simulink model "Nanogrid"  (R2026a)
settings: Solver=VariableStepAuto  StopTime=3
PreLoadFcn:
  | NanogridParam
undefined symbols (not defined in the file): baseLoad, bessSystem, bessVoltage, DiscIntNeverNeededParam, ee_sli_rtmsupport, gcbh, gflInverter, gfmInverter, nanoLoad, PV, PVInverter, ref, solar, solarInsolationChange, Ts
libraries: nesl_utility x51, eeGeneralControl x38, ee_lib x33, fl_lib x24, simulink x20, eeTransforms x13, slpidlib x8, nesl_utility_internal x4, sl_signal_attributes x4, sl_discontinuities x4, eeSinusoidalMeasurementV2 x3, batteryecm_lib x2
(part 4 of 6)

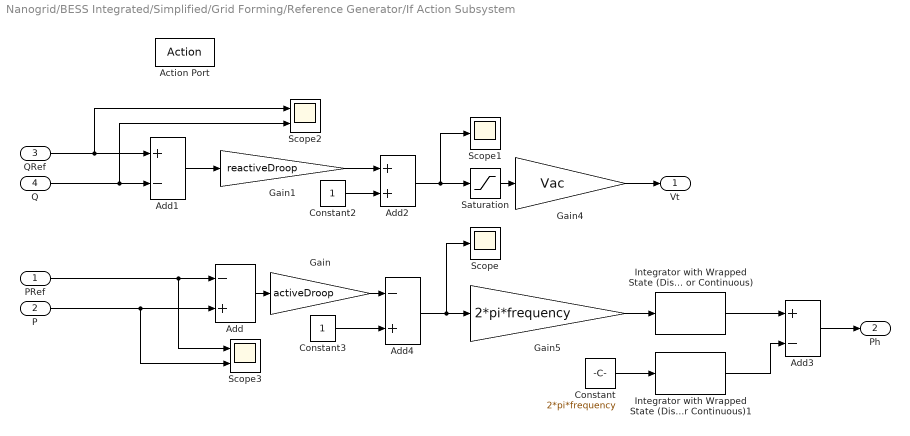
== system Nanogrid/BESS Integrated/Simplified/Grid Forming/Reference Generator/If Action Subsystem ==
  PRef : Inport
  P : Inport  Port=2
  QRef : Inport  Port=3
  Q : Inport  Port=4
  Action Port : ActionPort
  Add : Sum  Inputs=-+
  Add1 : Sum  Inputs=+-
  Add2 : Sum
  Add3 : Sum  Inputs=+-
  Add4 : Sum  Inputs=-+
  Constant : Constant  Value=2*pi*frequency  SampleTime=-1
  Constant2 : Constant
  Constant3 : Constant
  Gain : Gain  Gain=activeDroop
  Gain1 : Gain  Gain=reactiveDroop
  Gain4 : Gain  Gain=Vac
  Gain5 : Gain  Gain=2*pi*frequency
  Integrator with Wrapped State (Discrete or Continuous) : eeGeneralControl/Integrator with Wrapped State (Discrete or Continuous)  LabelModeActiveChoice=Discrete  WrappedStateUpperValue=2*pi  WrappedStateLowerValue=0  x0=0  Ts=-1
  Integrator with Wrapped State (Discrete or Continuous)1 : eeGeneralControl/Integrator with Wrapped State (Discrete or Continuous)  LabelModeActiveChoice=Discrete  WrappedStateUpperValue=2*pi  WrappedStateLowerValue=0  x0=0  Ts=-1
  Saturation : Saturate  UpperLimit=1.1  LowerLimit=0.9
  Scope : Scope
      settings: ActiveDisplayYMinimum=-1  ActiveDisplayYMaximum=1  DataLoggingVariableName=ScopeData2
  Scope1 : Scope
      settings: ActiveDisplayYMinimum=-1  ActiveDisplayYMaximum=1  DataLoggingVariableName=ScopeData3
  Scope2 : Scope  NumInputPorts=2
      settings: ActiveDisplayYMinimum=-1  ActiveDisplayYMaximum=1
  Scope3 : Scope  NumInputPorts=2
      settings: ActiveDisplayYMinimum=-1  ActiveDisplayYMaximum=1  DataLoggingVariableName=ScopeData2
  Vt : Outport
  Ph : Outport  Port=2
  wires:
  Add4/1 -> Scope/1, Gain5/1
  Gain/1 -> Add4/1
  Add1/1 -> Gain1/1
  Add2/1 -> Scope1/1, Saturation/1
  Gain5/1 -> Integrator with Wrapped State (Discrete or Continuous)/1
  Constant3/1 -> Add4/2
  Integrator with Wrapped State (Discrete or Continuous)/1 -> Add3/1
  Constant2/1 -> Add2/2
  Gain1/1 -> Add2/1
  Gain4/1 -> Vt/1
  QRef/1 -> Add1/1, Scope2/1
  Saturation/1 -> Gain4/1
  Add/1 -> Gain/1
  PRef/1 -> Add/1, Scope3/1
  Add3/1 -> Ph/1
  Constant/1 -> Integrator with Wrapped State (Discrete or Continuous)1/1
  Integrator with Wrapped State (Discrete or Continuous)1/1 -> Add3/2
  P/1 -> Add/2, Scope3/2
  Q/1 -> Add1/2, Scope2/2

== system Nanogrid/BESS Integrated/Simplified/Grid Forming/Reference Generator/If Action Subsystem1 ==
  PRef : Inport
  P : Inport  Port=2
  VRef : Inport  Port=3
  V : Inport  Port=4
  Action Port : ActionPort
  Add : Sum  Inputs=+-
  Add1 : Sum  Inputs=+-
  Add2 : Sum
  Add3 : Sum  Inputs=+-
  Add4 : Sum  Inputs=-+
  Constant2 : Constant
  Constant3 : Constant
  Constant4 : Constant  Value=0
  Gain : Gain  Gain=reactiveDroop
  Gain1 : Gain  Gain=activeDroop
  Gain4 : Gain  Gain=systemVoltage
  Gain5 : Gain  Gain=2*pi*systemFrequency
  Integrator with Wrapped State (Discrete or Continuous) : eeGeneralControl/Integrator with Wrapped State (Discrete or Continuous)  LabelModeActiveChoice=Discrete  WrappedStateUpperValue=2*pi  WrappedStateLowerValue=0  x0=0  Ts=-1
  Saturation : Saturate  UpperLimit=1.1  LowerLimit=0.9
  Vt : Outport
  Ph : Outport  Port=2
  wires:
  Add/1 -> Gain/1
  Constant4/1 -> Add3/2
  Add4/1 -> Gain5/1
  Gain/1 -> Add4/1
  Add1/1 -> Gain1/1
  Add2/1 -> Saturation/1
  Gain5/1 -> Integrator with Wrapped State (Discrete or Continuous)/1
  Constant3/1 -> Add4/2
  Integrator with Wrapped State (Discrete or Continuous)/1 -> Add3/1
  Constant2/1 -> Add2/2
  Gain1/1 -> Add2/1
  V/1 -> Add/2
  Gain4/1 -> Vt/1
  P/1 -> Add1/2
  VRef/1 -> Add/1
  PRef/1 -> Add1/1
  Add3/1 -> Ph/1
  Saturation/1 -> Gain4/1

== system Nanogrid/Solar Plant Integrated/Detailed/PV Plant & Controller/Controller/MPPT ==
  Qref : Inport
  ipv (A) : Inport  Port=2
  vdc (V) : Inport  Port=3
  Vabc : Inport  Port=4
  Iabc : Inport  Port=5
  Action Port : ActionPort  ActionPortLabel=if(u1 > 0)
  Solar PV Controller : Subsystem  LoadFcn=ee_sli_rtmsupport( 'loadfcn', gcbh );  mask(Solar PV Controller (Three-Phase)){L=filterInductance, frequency=frequency, iMax=iMaxPU, zBase=Vac^2/(plantRating*1000), mVAbase=plantRating*1000, VdcBase=baseVoltageDC, sampleTime=-1, Choice=Perturb and observe (P&O), Vdc=1100, delV=3, tSettling=1e-3, Kppll=100, Kipll=2000, initialPhase=0, Kpv=PV.controllerKpv, Kiv=PV.controllerKiv, Kdv=0, Kpicd=PV.controllerKpIc, Kiicd=PV.controllerKiIc, Kdicd=0, Kpicq=PV.controllerKpIc, Kiicq=PV.controllerKiIc, Kdicq=0}
      mask prompts: L "physmod:ee:library:comments:control:eeRenewablesControl:ACFilterInductanceH_MP"; frequency "physmod:ee:library:comments:control:eeRenewablesControl:SystemFrequencyHz_MP"; iMax "physmod:ee:library:comments:control:eeRenewablesControl:InverterCurrentLimitpu_MP"; zBase "physmod:ee:library:comments:control:eeRenewablesControl:BaseImpedanceACSideOhm_MP"; mVAbase "physmod:ee:library:comments:control:eeRenewablesControl:BaseMVA_MP"; VdcBase "physmod:ee:library:comments:control:eeRenewablesControl:DCBusBaseVoltageV_MP"; sampleTime "physmod:ee:library:comments:control:eeRenewablesControl:SampleTime1ForInherited_MP"; Choice "physmod:ee:library:comments:control:eeRenewablesControl:Algorithm_MP"; Vdc "physmod:ee:library:comments:control:eeRenewablesControl:InitialVoltageForMPPTV_MP"; delV "physmod:ee:library:comments:control:eeRenewablesControl:VoltageStepOfMPPTV_MP"; tSettling "physmod:ee:library:comments:control:eeRenewablesControl:SettlingTimeOfMPPTs_MP"; Kppll "physmod:ee:library:comments:control:eeRenewablesControl:ProportionalGain_MP"; Kipll "physmod:ee:library:comments:control:eeRenewablesControl:IntegralGain_MP"; initialPhase "physmod:ee:library:comments:control:eeRenewablesControl:InitialPhaseAngle_MP"; Kpv "physmod:ee:library:comments:control:eeRenewablesControl:ProportionalGain_MP"; Kiv "physmod:ee:library:comments:control:eeRenewablesControl:IntegralGain_MP"; Kdv "physmod:ee:library:comments:control:eeRenewablesControl:DerivativeGain_MP"; Kpicd "physmod:ee:library:comments:control:eeRenewablesControl:DaxisProportionalGain_MP"; Kiicd "physmod:ee:library:comments:control:eeRenewablesControl:DaxisIntegralGain_MP"; Kdicd "physmod:ee:library:comments:control:eeRenewablesControl:DaxisDerivativeGain_MP"; Kpicq "physmod:ee:library:comments:control:eeRenewablesControl:QaxisProportionalGain_MP"; Kiicq "physmod:ee:library:comments:control:eeRenewablesControl:QaxisIntegralGain_MP"; Kdicq "physmod:ee:library:comments:control:eeRenewablesControl:QaxisDerivativeGain_MP"
      mask help: physmod:ee:library:comments:control:eeRenewablesControl:PVGridFollowingController_MD
      mask init:
      | timeDomain = ee.mask.getSampleTimeDomain(sampleTime,gcb);
      | if sampleTime < 0 && sampleTime ~= -1            
      |     error(message('physmod:ee:library:MinusOneZeroOrPositive',getString(message('physmod:ee:library:comments:control:eeRenewablesControl:SampleTime1ForInherited_MP'))));            
      | end
      | if L <= 0            
      |     error(message('physmod:simscape:compiler:patterns:checks:GreaterThanZero',getString(message('physmod:ee:library:comments:control:eeRenewablesControl:ACFilterInductanceH_MP'))));            
      | end
      | if VdcBase <= 0            
      |     error(message('physmod:simscape:compiler:patterns:checks:GreaterThanZero',getString(message('physmod:ee:library:comments:control:eeRenewablesControl:DCBusBaseVoltageV_MP'))));            
      | end
      | if delV <= 0            
      |     error(message('physmod:simscape:compiler:patterns:checks:GreaterThanZero',getString(message('physmod:ee:library:comments:control:eeRenewablesControl:VoltageStepOfMPPTV_MP'))));            
      | end
      | if tSettling <= 0            
      |     error(message('physmod:simscape:compiler:patterns:checks:GreaterThanZero',getString(message('physmod:ee:library:comments:control:eeRenewablesControl:SettlingTimeOfMPPTs_MP'))));            
      | end
      | if zBase <= 0            
      |     error(message('physmod:simscape:compiler:patterns:checks:GreaterThanZero',getString(message('physmod:ee:library:comments:control:eeRenewablesControl:BaseImpedanceACSideOhm_MP'))));            
      | end
      | if iMax <= 0            
      |     error(message('physmod:simscape:compiler:patterns:checks:GreaterThanZero',getString(message('physmod:ee:library:comments:control:eeRenewablesControl:InverterCurrentLimitpu_MP'))));            
      | end
      | if frequency <= 0            
      |     error(message('physmod:simscape:compiler:patterns:checks:GreaterThanZero',getString(message('physmod:ee:library:comments:control:eeRenewablesControl:SystemFrequencyHz_MP'))));            
      | end
      settings: CopyFcn=ee_sli_rtmsupport( 'copyfcn', gcbh );  DeleteFcn=ee_sli_rtmsupport( 'deletefcn', gcbh );  ModelCloseFcn=ee_sli_rtmsupport( 'modelclosefcn', gcbh );  PostSaveFcn=ee_sli_rtmsupport( 'postsavefcn', gcbh );  PreCopyFcn=ee_sli_rtmsupport( 'precopyfcn', gcbh );  OpenFcn=ee_sli_rtmsupport( 'openfcn', gcbh );  CloseFcn=ee_sli_rtmsupport( 'closefcn', gcbh );  PreDeleteFcn=ee_sli_rtmsupport( 'predeletefcn', gcbh );
      mask Help: web(nesl_help(gcbh))
      mask TypeOptions sampleTime: Current_controller/SystemSampleTime | DC voltage controller & current reference/SystemSampleTime
      mask TypeOptions Choice: Variant Subsystem/LabelModeActiveChoice
      mask DialogControl Container4 Prompt: physmod:ee:library:comments:control:eeRenewablesControl:General_Tab
      mask DialogControl L Prompt: AC filter inductance (H)
      mask DialogControl frequency Prompt: System frequency (Hz)
      mask DialogControl iMax Prompt: Inverter current limit (pu)
      mask DialogControl zBase Prompt: Base impedance on AC side (Ohm)
      mask DialogControl mVAbase Prompt: Base power on AC side (V*A)
      mask DialogControl VdcBase Prompt: DC bus base voltage (V)
      mask DialogControl sampleTime Prompt: Sample time (-1 for inherited)
      mask DialogControl Container5 Prompt: physmod:ee:library:comments:control:eeRenewablesControl:MPPT_Tab
      mask DialogControl Choice Prompt: Algorithm
      mask DialogControl Vdc Prompt: Initial voltage for MPPT (V)
      mask DialogControl delV Prompt: Voltage step of MPPT (V)
      mask DialogControl tSettling Prompt: Settling time of MPPT (s)
      mask DialogControl Container6 Prompt: physmod:ee:library:comments:control:eeRenewablesControl:PLL_Tab
      mask DialogControl Kppll Prompt: Proportional gain
      mask DialogControl Kipll Prompt: Integral gain
      mask DialogControl initialPhase Prompt: Initial phase angle (deg)
      mask DialogControl Container7 Prompt: physmod:ee:library:comments:control:eeRenewablesControl:VoltageController_Tab
      mask DialogControl Kpv Prompt: Proportional gain
      mask DialogControl Kiv Prompt: Integral gain
      mask DialogControl Kdv Prompt: Derivative gain
      mask DialogControl Container8 Prompt: physmod:ee:library:comments:control:eeRenewablesControl:CurrentController_Tab
      mask DialogControl Kpicd Prompt: D-axis proportional gain
      mask DialogControl Kiicd Prompt: D-axis integral gain
      mask DialogControl Kdicd Prompt: D-axis derivative gain
      mask DialogControl Kpicq Prompt: Q-axis proportional gain
      mask DialogControl Kiicq Prompt: Q-axis integral gain
      mask DialogControl Kdicq Prompt: Q-axis derivative gain
      mask Display: ee.mask.drawPVcontroller;
  mabc : Outport
  wires:
  ipv (A)/1 -> Solar PV Controller/2(ipv (A))
  Iabc/1 -> Solar PV Controller/5(iabc (pu))
  Vabc/1 -> Solar PV Controller/4(vabc (pu))
  vdc (V)/1 -> Solar PV Controller/3(vdc (V))
  Qref/1 -> Solar PV Controller/1(Qref (pu))
  Solar PV Controller/1(vabcRef (pu)) -> mabc/1

== system Nanogrid/Solar Plant Integrated/Detailed/PV Plant & Controller/Controller/Power Reference ==
  Iabc : Inport
  Vabc : Inport  Port=2
  PRef : Inport  Port=3
  QRef : Inport  Port=4
  Action Port : ActionPort  ActionPortLabel=else
  Power Reference Controller : Subsystem  mask(Power Reference Controller){frequency=frequency, P=Real power, MVA=plantRating*1000, zbase=Vac^2/plantRating, L=filterInductance, Imax=iMaxPU, Td=1e-3, Kpic=1.5, Kiic=10, Kd=0, kpPLL=40, kiPLL=1000, kdPLL=0}
      mask prompts: frequency "Frequency (Hz)"; P "Priority mode"; MVA "Base Power (V*A)"; zbase "Base Impedance (Ohm)"; L "Filter Inductance (H)"; Imax "Inverter current limit (pu)"; Td "Sensor time delay (s)"; Kpic "Proportional gain"; Kiic "Integral gain"; Kd "Derevative gain"; kpPLL "Proportional gain"; kiPLL "Integral gain"; kdPLL "Derevative gain"
      mask help: This block receives active and reactive power references for the converter based on system requirements or higher-level control commands. It ensures that the converter operates according to desired power setpoints, supporting grid services such as frequency regulation, voltage support, and power dispatch
      settings: CopyFcn=set_param(gcbh,'LinkStatus','none');
      mask TypeOptions P: Real power  | Reactive power
      mask DialogControl Container4 Prompt: General
      mask DialogControl Container5 Prompt: Current Controller
      mask DialogControl Container5_copy Prompt: PLL
  mabc : Outport
  wires:
  QRef/1 -> Power Reference Controller/4(Qref)
  PRef/1 -> Power Reference Controller/3(Pref)
  Power Reference Controller/1(mabc) -> mabc/1
  Vabc/1 -> Power Reference Controller/2(Vabc)
  Iabc/1 -> Power Reference Controller/1(Iabc)

== system Nanogrid/Solar Plant Integrated/Detailed/PV Plant & Controller/PV Plant/Converter ==
  mabc : Inport
  Average : Subsystem  VariantControl=Average
  Switching : Subsystem  VariantControl=Switching
  + : PMIOPort  Side=Left
  - : PMIOPort  Port=2  Side=Left
  ~ : PMIOPort  Port=3  Side=Right

== system Nanogrid/Solar Plant Integrated/Detailed/PV Plant & Controller/Sensor Dynamics/Current Measurement ==
  u : Inport
  Lead-Lag (Discrete or Continuous) : eeGeneralControl/Lead-Lag (Discrete or Continuous)  T1=0  T2=PV.controllerTSensor  B=inf  A=-inf  init_option=Inherited from block input  x0=0  Ts=Ts
  V : Outport
  wires:
  u/1 -> Lead-Lag (Discrete or Continuous)/1
  Lead-Lag (Discrete or Continuous)/1 -> V/1

== system Nanogrid/Solar Plant Integrated/Detailed/PV Plant & Controller/Sensor Dynamics/Voltage Measurement ==
  u : Inport
  Lead-Lag (Discrete or Continuous) : eeGeneralControl/Lead-Lag (Discrete or Continuous)  T1=0  T2=PV.controllerTSensor  B=inf  A=-inf  init_option=Inherited from block input  x0=0  Ts=Ts
  I : Outport
  wires:
  u/1 -> Lead-Lag (Discrete or Continuous)/1
  Lead-Lag (Discrete or Continuous)/1 -> I/1

== system Nanogrid/BESS Integrated/Detailed/BESS Controller/Grid Following/Reference Current/Current limits ==
  Imax : Inport
  iqref : Inport  Port=2
  idref : Inport  Port=3
  Constant8 : Constant  Value=0
  Constant9 : Constant  Value=0
  Scope : Scope
      settings: ActiveDisplayYMinimum=-0.14399  ActiveDisplayYMaximum=1.29587  DataLoggingVariableName=ScopeData3
  Scope1 : Scope
      settings: ActiveDisplayYMinimum=-0.13655  ActiveDisplayYMaximum=1.22893  DataLoggingVariableName=ScopeData4
  Sqrt : Sqrt
  Sqrt1 : Sqrt
  Square{1..4} (4 alike) : Math  Operator=square
  Step2 : Step  Time=0.01  SampleTime=Ts
  Step3 : Step  Time=0.01  SampleTime=Ts
  Sum6 : Sum  Inputs=|+-
  Sum9 : Sum  Inputs=|+-
  Switch1 : Switch  Threshold=.01  SaturateOnIntegerOverflow=off  InputSameDT=off
  Switch2 : Switch  Threshold=.01  SaturateOnIntegerOverflow=off  InputSameDT=off
  iubq : Outport
  iubd : Outport  Port=2
  wires:
  idref/1 -> Square4/1
  Sqrt1/1 -> iubq/1, Scope1/1
  Imax/1 -> Square1/1, Square3/1
  Sqrt/1 -> iubd/1, Scope/1
  Constant9/1 -> Switch2/3
  Square4/1 -> Sum9/2
  Constant8/1 -> Switch1/3
  Square2/1 -> Sum6/2
  Sum6/1 -> Switch1/1
  Square3/1 -> Sum9/1
  iqref/1 -> Square2/1
  Switch1/1 -> Sqrt/1
  Square1/1 -> Sum6/1
  Switch2/1 -> Sqrt1/1
  Step2/1 -> Switch1/2
  Step3/1 -> Switch2/2
  Sum9/1 -> Switch2/1

== system Nanogrid/BESS Integrated/Detailed/BESS Controller/Grid Following/Reference Current/Refernce id generation ==
  V_mag : Inport
  del f : Inport  Port=2
  ubid : Inport  Port=3
  PRef : Inport  Port=4
  Divide : Product  Inputs=/*
  Gain6 : Gain  Gain=-1
  P/Q Priority : Switch  Criteria=u2 ~= 0  SaturateOnIntegerOverflow=off  InputSameDT=off
  Priority Mode : Constant  Value=P-2
  Saturation Dynamic2 : simulink/Discontinuities/Saturation Dynamic  OutMin=[]  OutMax=[]  OutDataTypeStr=Inherit: Same as second input  OutDataType=fixdt(1, 16)  OutScaling=2^-10  DoSatur=off
  Saturation1 : Saturate  UpperLimit=Imax  LowerLimit=-Imax
  Scope : Scope
      settings: ActiveDisplayYMinimum=-1  ActiveDisplayYMaximum=1
  Scope1 : Scope
      settings: ActiveDisplayYMinimum=-0.68622  ActiveDisplayYMaximum=0.07625  DataLoggingVariableName=ScopeData2
  Sum : Sum  Inputs=|++
  droop m_p : Gain  Gain=mp/MVA
  ubid1 : InportShadow  Port=3
  id_ref : Outport
  wires:
  del f/1 -> droop m_p/1
  Divide/1 -> Saturation Dynamic2/2, Saturation1/1
  V_mag/1 -> Divide/1
  P/Q Priority/1 -> id_ref/1, Scope/1
  ubid1/1 -> Gain6/1
  Saturation1/1 -> P/Q Priority/1
  Priority Mode/1 -> P/Q Priority/2
  PRef/1 -> Sum/2
  Saturation Dynamic2/1 -> P/Q Priority/3, Scope1/1
  Gain6/1 -> Saturation Dynamic2/3
  ubid/1 -> Saturation Dynamic2/1
  Sum/1 -> Divide/2
  droop m_p/1 -> Sum/1

== system Nanogrid/BESS Integrated/Detailed/BESS Controller/Grid Following/Reference Current/Refernce iq generation ==
  ubiq : Inport
  V_ref : Inport  Port=2
  V_mag : Inport  Port=3
  LVRT_iq : Inport  Port=4
  Q_ref : Inport  Port=5
  Divide1 : Product  Inputs=*/
  Gain : Gain  Gain=-1
  Gain1 : Gain  Gain=-1
  Gain7 : Gain  Gain=-1
  LVRT Priority : Switch  Threshold=.9  SaturateOnIntegerOverflow=off  InputSameDT=off
  P/Q Priority : Switch  Criteria=u2 ~= 0  SaturateOnIntegerOverflow=off  InputSameDT=off
  Priority Mode : Constant  Value=P-2
  Saturation Dynamic : simulink/Discontinuities/Saturation Dynamic  OutMin=[]  OutMax=[]  OutDataTypeStr=Inherit: Same as second input  OutDataType=fixdt(1, 16)  OutScaling=2^-10  DoSatur=off
  Saturation2 : Saturate  UpperLimit=1  LowerLimit=-1
  Saturation3 : Saturate  UpperLimit=Imax  LowerLimit=-Imax
  Sum : Sum  Inputs=|++
  Sum1 : Sum  Inputs=|-+
  droop m_v : Gain  Gain=mv
  ubiq1 : InportShadow
  iq_ref : Outport
  wires:
  Gain/1 -> iq_ref/1
  V_mag/1 -> Sum1/2, Divide1/2, LVRT Priority/2
  Q_ref/1 -> Sum/1
  Sum/1 -> Divide1/1
  droop m_v/1 -> Sum/2
  ubiq1/1 -> Gain7/1
  LVRT_iq/1 -> Saturation2/1
  V_ref/1 -> Sum1/1
  Gain7/1 -> Saturation Dynamic/3
  Saturation Dynamic/1 -> P/Q Priority/1
  Divide1/1 -> Saturation3/1, Saturation Dynamic/2
  Priority Mode/1 -> P/Q Priority/2
  Saturation3/1 -> P/Q Priority/3
  Saturation2/1 -> Gain1/1
  ubiq/1 -> Saturation Dynamic/1
  Gain1/1 -> LVRT Priority/3
  P/Q Priority/1 -> LVRT Priority/1
  Sum1/1 -> droop m_v/1
  LVRT Priority/1 -> Gain/1

== system Nanogrid/BESS Integrated/Detailed/BESS Controller/Grid Forming/Current Limiting/CurrentLimitingMethod ==
  Igd : Inport
  Igq : Inport  Port=2
  currentLimitAndVirtual : Subsystem  VariantControl=both
  currentSaturation : Subsystem  VariantControl=ctSat
  virtualImpedance : Subsystem  VariantControl=virimp
  delVd : Outport
  delVq : Outport  Port=2
  Idmax : Outport  Port=3
  Iqmax : Outport  Port=4

== system Nanogrid/BESS Integrated/Detailed/BESS Controller/Grid Forming/Grid Voltage Reactive Power Support/Modifying Active Power Reference ==
  PrefInput : Inport
  Vd : Inport  Port=2
  Igd : Inport  Port=3
  Igq : Inport  Port=4
  AND : Logic  IconShape=distinctive  AllPortsSameDT=off  OutDataTypeStr=boolean
  Abs : Abs  SaturateOnIntegerOverflow=off
  Compare To Constant : simulink/Logic and Bit Operations/Compare To Constant  relop=>=  const=0.95  OutDataTypeStr=boolean
  Computing New Active Power Ref : Subsystem
  Math Function1 : Math  Operator=hypot
  Power Sign : Signum
  Product : Product
  Relay : Relay  OnSwitchValue=40%maxVICurrentLimit*0.96  OffSwitchValue=1
  Scope : Scope
  Scope1 : Scope
  Scope2 : Scope
  Switch : Switch  Criteria=u2 > Threshold  SaturateOnIntegerOverflow=off  InputSameDT=off
  Pref : Outport
  wires:
  Compare To Constant/1 -> AND/1
  AND/1 -> Switch/2
  Relay/1 -> AND/2, Scope1/1
  Product/1 -> Pref/1
  Power Sign/1 -> Product/2
  Abs/1 -> Product/1
  Switch/1 -> Abs/1
  Igq/1 -> Math Function1/1, Computing New Active Power Ref/1(Iq)
  Igd/1 -> Math Function1/2
  PrefInput/1 -> Switch/3, Power Sign/1
  Vd/1 -> Compare To Constant/1, Computing New Active Power Ref/2(Vd)
  Math Function1/1 -> Relay/1, Scope2/1  "Is"
  Computing New Active Power Ref/1(Pref) -> Scope/1, Switch/1

== system Nanogrid/BESS Integrated/Detailed/BESS Controller/Grid Forming/Grid Voltage Reactive Power Support/Modifying Reactive Power Reference ==
  Vgd : Inport
  Vgq : Inport  Port=2
  Qref : Inport  Port=3
  Pref : Inport  Port=4
  Changing the Power Reference : Subsystem
  Hysteresis : Subsystem
  Math Function : Math  Operator=hypot
  Merge : Merge
  Merge1 : Merge
  NOT : Logic  Operator=NOT  IconShape=distinctive  AllPortsSameDT=off  OutDataTypeStr=boolean
  Not Altering the Power Reference : Subsystem
  Scope : Scope
  PrefNew : Outport
  QrefNew : Outport  Port=2
  wires:
  [Qref] -> Changing the Power Reference/4(Qref)
  [Pref] -> Changing the Power Reference/3(Pref)
  Merge/1 -> PrefNew/1
  Merge1/1 -> QrefNew/1
  Pref/1 -> [Pref], Not Altering the Power Reference/1(Pref)
  Vgq/1 -> Math Function/2
  Changing the Power Reference/2(Qrefv) -> Merge1/1
  [Vd] -> Changing the Power Reference/2(Vd)
  Hysteresis/1(LVFlag) -> NOT/1, Changing the Power Reference/Enable, Scope/1
  Qref/1 -> [Qref], Not Altering the Power Reference/2(Qref)
  NOT/1 -> Not Altering the Power Reference/Enable
  Changing the Power Reference/1(Prefv) -> Merge/1
  Not Altering the Power Reference/1(Prefv) -> Merge/2
  [Vs] -> Changing the Power Reference/1(Vs)
  Math Function/1 -> [Vs], Hysteresis/1(Vs)
  Not Altering the Power Reference/2(Qrefv) -> Merge1/2
  Vgd/1 -> Math Function/1, [Vd]

== system Nanogrid/BESS Integrated/Detailed/BESS Controller/Grid Forming/Measurement/Frequency Measurement ==
  Vabc : Inport
  Convert To PU : Gain  Gain=1/powerFreq
  Frequency Measurement : Subsystem  TreatAsAtomicUnit=on  SystemSampleTime=sampleTime  mask{initialFrequency=powerFreq, sampleTime=activePowerSampleTime}
      mask prompts: initialFrequency "Initial frequency in Hz"; sampleTime "Sample time in sec"
      mask DialogControl Container7 Prompt: General
  Low-Pass Filter : eeGeneralControl/Low-Pass Filter (Discrete or Continuous)  K=1  T=freqMeasTimeConst  B=inf  A=-inf  init_option=Inherited from block input  x0=0  Ts=-1
  freq : Outport
  wires:
  Vabc/1 -> Frequency Measurement/1(abc)
  Convert To PU/1 -> freq/1
  Frequency Measurement/1(Freq) -> Low-Pass Filter/1
  Low-Pass Filter/1 -> Convert To PU/1  "Freq"

== system Nanogrid/BESS Integrated/Detailed/BESS Controller/Grid Forming/Measurement/abc2dq ==
  Igabc : Inport
  Angle : Inport  Port=2
  Vgabc : Inport  Port=3
  Supply Current to dq : Subsystem
  Supply Voltage  to dq1 : Subsystem
  Vgd : Outport
  Vgq : Outport  Port=2
  Igd : Outport  Port=3
  Igq : Outport  Port=4
  wires:
  Supply Voltage  to dq1/2(Vgq) -> Vgq/1  "Vgq"
  Supply Voltage  to dq1/1(Vgd) -> Vgd/1  "Vgd"
  Supply Current to dq/2(Igq) -> Igq/1  "Iq"
  Supply Current to dq/1(Igd) -> Igd/1  "Id"
  Igabc/1 -> Supply Current to dq/1(abc)
  Vgabc/1 -> Supply Voltage  to dq1/2(abc)
  Angle/1 -> Supply Current to dq/2(Angle), Supply Voltage  to dq1/1(Angle)

== system Nanogrid/BESS Integrated/Detailed/BESS Controller/Grid Forming/Power Control/ActivePowerControl ==
  Pref : Inport
  Pmeas : Inport  Port=2
  fref : Inport  Port=3
  cntrlflag : Inport  Port=4
  fgrid : Inport  Port=5
  droopControl : Subsystem  VariantControl=droop
  vsmControl : Subsystem  VariantControl=vsm
  Theta : Outport
  w : Outport  Port=2

== system Nanogrid/BESS Integrated/Detailed/BESS Controller/Grid Forming/Power Control/ReactiveControl ==
  note: Vs-delV
  CntrlFlag : Inport
  Qref : Inport  Port=2
  Qmeas : Inport  Port=3
  Vgdmeas : Inport  Port=4
  Vref : Inport  Port=5
  Constant2 : Constant  Value=0
  Saturation1 : Saturate  UpperLimit=(dcBusVoltage/2)/(sqrt(2/3)*girdLineVoltage)  LowerLimit=-(dcBusVoltage/2)/(sqrt(2/3)*girdLineVoltage)
  Scope : Scope
      settings: ActiveDisplayYMinimum=-1  ActiveDisplayYMaximum=1  DataLoggingVariableName=ScopeData20
  Voltage  Reference Selection : Subsystem
  Vmd : Outport
  Vmq : Outport  Port=2
  wires:
  Vgdmeas/1 -> Voltage  Reference Selection/5(Vgdmeas)
  Vref/1 -> Voltage  Reference Selection/4(Vref)
  Qmeas/1 -> Voltage  Reference Selection/3(Qmeas)
  Qref/1 -> Voltage  Reference Selection/2(Qref)
  CntrlFlag/1 -> Voltage  Reference Selection/1(cntrlflag)
  Saturation1/1 -> Vmd/1, Scope/1
  Constant2/1 -> Vmq/1
  Voltage  Reference Selection/1(Vd) -> Saturation1/1  "Q"

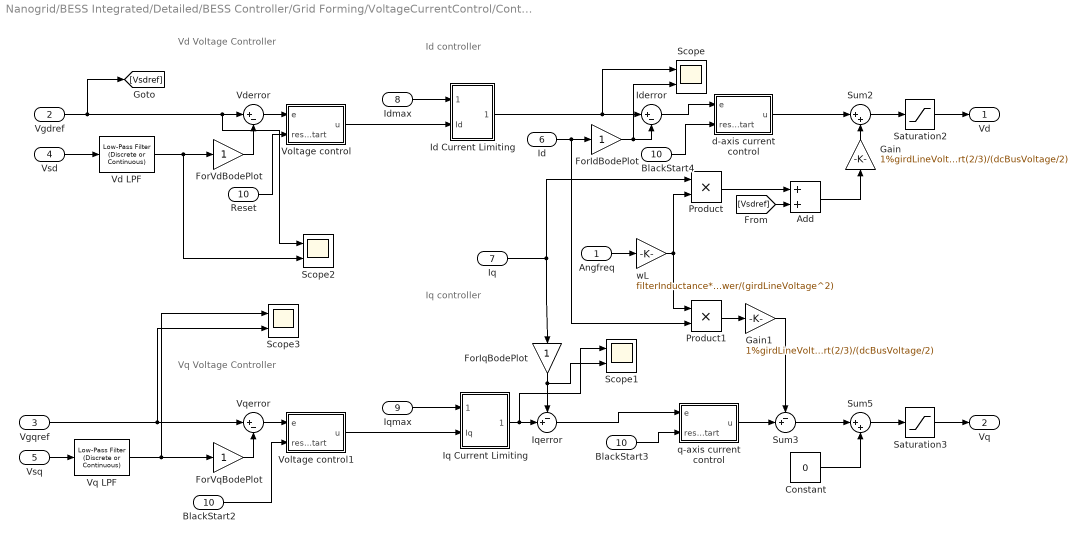
== system Nanogrid/BESS Integrated/Detailed/BESS Controller/Grid Forming/VoltageCurrentControl/Controller ==
  note: Vq Voltage Controller
  note: Iq controller
  note: Vd Voltage Controller
  note: Id controller
  Angfreq : Inport
  Vgdref : Inport  Port=2
  Vgqref : Inport  Port=3
  Vsd : Inport  Port=4
  Vsq : Inport  Port=5
  Id : Inport  Port=6
  Iq : Inport  Port=7
  Idmax : Inport  Port=8
  Iqmax : Inport  Port=9
  Reset : Inport  Port=10
  Add : Sum
  BlackStart2 : InportShadow  Port=10
  BlackStart3 : InportShadow  Port=10
  BlackStart4 : InportShadow  Port=10
  Constant : Constant  Value=0  SampleTime=currentControlTs
  ForIdBodePlot : Gain
  ForIqBodePlot : Gain
  ForVdBodePlot : Gain
  ForVqBodePlot : Gain
  Gain : Gain  Gain=1%girdLineVoltage*sqrt(2/3)/(dcBusVoltage/2)
  Gain1 : Gain  Gain=1%girdLineVoltage*sqrt(2/3)/(dcBusVoltage/2)
  Id Current Limiting : Subsystem
  Iderror : Sum  Inputs=|+-
  Iq Current Limiting : Subsystem
  Iqerror : Sum  Inputs=-+|
  Product : Product
  Product1 : Product
  Saturation2 : Saturate  UpperLimit=4  LowerLimit=-3
  Saturation3 : Saturate  UpperLimit=3  LowerLimit=-3
  Scope{,1..3} (4 alike) : Scope  NumInputPorts=2
      Scope settings: ActiveDisplayYMinimum=-0.33488  ActiveDisplayYMaximum=2.03721
      Scope2 settings: ActiveDisplayYMinimum=-0.14129  ActiveDisplayYMaximum=1.2716
  Sum2 : Sum  Inputs=|++
  Sum3 : Sum  Inputs=-+|
  Sum5 : Sum  Inputs=|++
  Vd LPF : eeGeneralControl/Low-Pass Filter (Discrete or Continuous)  K=1  T=vdvqLPFTimeConst  B=inf  A=-inf  init_option=Specify as parameter  x0=0  Ts=voltControlTs
  Vderror : Sum  Inputs=|+-
  Voltage control : Subsystem
  Voltage control1 : Subsystem
  Vq LPF : eeGeneralControl/Low-Pass Filter (Discrete or Continuous)  K=1  T=vdvqLPFTimeConst  B=inf  A=-inf  init_option=Inherited from block input  x0=0  Ts=voltControlTs
  Vqerror : Sum  Inputs=|+-
  d-axis current control : Subsystem
  q-axis current control : Subsystem
  wL : Gain  Gain=filterInductance*power/(girdLineVoltage^2)
  Vd : Outport  VectorParamsAs1DForOutWhenUnconnected=off
  Vq : Outport  Port=2  VectorParamsAs1DForOutWhenUnconnected=off
  wires:
  Vgdref/1 -> [Vsdref], Vderror/1, Scope2/1
  BlackStart4/1 -> d-axis current control/2(resetBlackStart)
  BlackStart3/1 -> q-axis current control/2(resetBlackStart)
  BlackStart2/1 -> Voltage control1/2(resetBlackStart)
  Reset/1 -> Voltage control/2(resetBlackStart)
  Vq LPF/1 -> ForVqBodePlot/1, Scope3/1
  Vd LPF/1 -> ForVdBodePlot/1, Scope2/2
  Id Current Limiting/1(Idref) -> Iderror/1, Scope/1
  ForIqBodePlot/1 -> Iqerror/1, Scope1/2
  ForIdBodePlot/1 -> Iderror/2, Scope/2
  ForVqBodePlot/1 -> Vqerror/2
  ForVdBodePlot/1 -> Vderror/2
  Vsd/1 -> Vd LPF/1
  Voltage control1/1(u) -> Iq Current Limiting/2(Iq)
  Iq Current Limiting/1(Iqref) -> Iqerror/2, Scope1/1
  Idmax/1 -> Id Current Limiting/1(Imax)
  Voltage control/1(u) -> Id Current Limiting/2(Id)
  Gain/1 -> Sum2/2
  Add/1 -> Gain/1
  [Vsdref] -> Add/2
  Gain1/1 -> Sum3/1
  Vqerror/1 -> Voltage control1/1(e)
  Vgqref/1 -> Vqerror/1, Scope3/2
  Iqmax/1 -> Iq Current Limiting/1(Imax)
  Vderror/1 -> Voltage control/1(e)
  Id/1 -> ForIdBodePlot/1, Product1/2
  Vsq/1 -> Vq LPF/1
  Sum5/1 -> Saturation3/1
  Sum3/1 -> Sum5/1
  q-axis current control/1(u) -> Sum3/2
  Sum2/1 -> Saturation2/1
  d-axis current control/1(u) -> Sum2/1
  Product/1 -> Add/1
  Product1/1 -> Gain1/1
  Saturation2/1 -> Vd/1
  Saturation3/1 -> Vq/1
  Iderror/1 -> d-axis current control/1(e)
  Constant/1 -> Sum5/2
  Angfreq/1 -> wL/1
  Iq/1 -> Product/1, ForIqBodePlot/1
  wL/1 -> Product/2, Product1/1
  Iqerror/1 -> q-axis current control/1(e)

== system Nanogrid/BESS Integrated/Detailed/BESS Controller/Grid Forming/VoltageCurrentControl/Modulation Signal ==
  Vd : Inport
  Vq : Inport  Port=2
  Angle : Inport  Port=3
  Constant : Constant  Value=0
  Inverse Park Transform : eeTransforms/Inverse Park Transform  AxisAlignment=D-axis  PowerInvariant=off
  Mux1 : Mux  Inputs=3
  Saturation2 : Saturate  UpperLimit=1  LowerLimit=-1
  Scope : Scope  NumInputPorts=2
      settings: DataLoggingVariableName=ScopeData9
  Scope1 : Scope
  mabc : Outport  VectorParamsAs1DForOutWhenUnconnected=off
  wires:
  Vq/1 -> Mux1/2, Scope/2
  Vd/1 -> Mux1/1, Scope/1
  Constant/1 -> Mux1/3
  Saturation2/1 -> mabc/1
  Angle/1 -> Inverse Park Transform/2, Scope1/1
  Mux1/1 -> Inverse Park Transform/1
  Inverse Park Transform/1 -> Saturation2/1

== system Nanogrid/BESS Integrated/Detailed/BESS Plant/Converter/Switching/Pulse Generation ==
  G : Inport
  Constant : Constant  Value=5
  Subtract : Sum  Inputs=-+
  G1 : Outport  VectorParamsAs1DForOutWhenUnconnected=off
  G2 : Outport  Port=2  VectorParamsAs1DForOutWhenUnconnected=off
  wires:
  G/1 -> Subtract/1, G1/1
  Constant/1 -> Subtract/2
  Subtract/1 -> G2/1

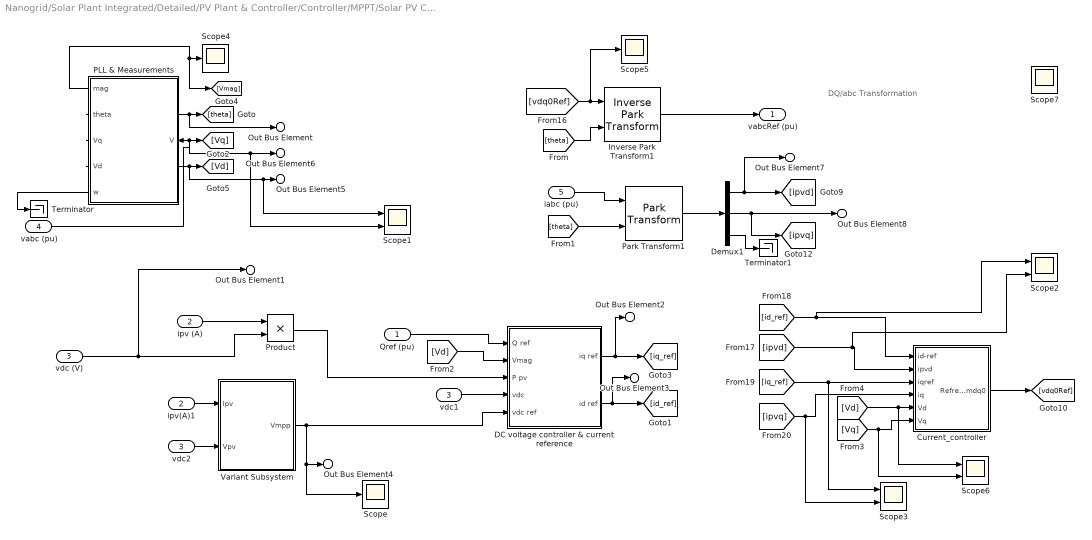
== system Nanogrid/Solar Plant Integrated/Detailed/PV Plant & Controller/Controller/MPPT/Solar PV Controller ==
  note: DQ/abc Transformation
  Qref (pu) : Inport
  ipv (A) : Inport  Port=2
  vdc (V) : Inport  Port=3
  vabc (pu) : Inport  Port=4
  iabc (pu) : Inport  Port=5
  Current_controller : Subsystem  SystemSampleTime=sampleTime
  DC voltage controller & current reference : Subsystem  SystemSampleTime=sampleTime
  Demux1 : Demux  Outputs=3
  Inverse Park Transform1 : eeTransforms/Inverse Park Transform  AxisAlignment=Q-axis  PowerInvariant=off
  PLL & Measurements : Subsystem
  Park Transform1 : eeTransforms/Park Transform  AxisAlignment=Q-axis  PowerInvariant=off
  Product : Product
  Scope{,4..5,7} (4 alike) : Scope
      Scope settings: ActiveDisplayYMinimum=719.47133  ActiveDisplayYMaximum=1441.72759  DataLoggingVariableName=ScopeData5
      Scope4 settings: ActiveDisplayYMinimum=-1  ActiveDisplayYMaximum=1
      Scope5 settings: ActiveDisplayYMinimum=-1  ActiveDisplayYMaximum=1
      Scope7 settings: DataLoggingVariableName=ScopeData43
  Scope{1..3,6} (4 alike) : Scope  NumInputPorts=2
      Scope1 settings: ActiveDisplayYMinimum=-0.005645300550064819  ActiveDisplayYMaximum=1.3041540601269743  DataLoggingVariableName=ScopeData6
      Scope2 settings: ActiveDisplayYMinimum=-0.14999999999999997  ActiveDisplayYMaximum=1.3499999999999999
      Scope3 settings: ActiveDisplayYMinimum=-0.016333965026179058  ActiveDisplayYMaximum=0.0079163760872077091
      Scope6 settings: ActiveDisplayYMinimum=-1  ActiveDisplayYMaximum=1  DataLoggingVariableName=ScopeData6
  Terminator : Terminator
  Terminator1 : Terminator
  Variant Subsystem : Subsystem  Variant=on  VariantControlMode=label  LabelModeActiveChoice=Perturb and observe (P&O)
  ipv(A)1 : InportShadow  Port=2
  vdc1 : InportShadow  Port=3
  vdc2 : InportShadow  Port=3
  vabcRef (pu) : Outport
  Out Bus Element : Outport  Port=2  PortName=visualization  Element=theta [rad]
  Out Bus Element1 : Outport  Port=2  PortName=visualization  Element=vdc [Volts]
  Out Bus Element2 : Outport  Port=2  PortName=visualization  Element=iq ref [pu]
  Out Bus Element3 : Outport  Port=2  PortName=visualization  Element=id ref [pu]
  Out Bus Element4 : Outport  Port=2  PortName=visualization  Element=vdc ref [Volts]
  Out Bus Element5 : Outport  Port=2  PortName=visualization  Element=Vd [pu]
  Out Bus Element6 : Outport  Port=2  PortName=visualization  Element=Vq [pu]
  Out Bus Element7 : Outport  Port=2  PortName=visualization  Element=id [pu]
  Out Bus Element8 : Outport  Port=2  PortName=visualization  Element=iq [pu]
  wires:
  PLL & Measurements/2(theta) -> [theta], Out Bus Element/1
  ipv(A)1/1 -> Variant Subsystem/1(Ipv)
  vdc2/1 -> Variant Subsystem/2(Vpv)
  ipv (A)/1 -> Product/1
  PLL & Measurements/5(w) -> Terminator/1
  Variant Subsystem/1(Vmpp) -> DC voltage controller & current reference/5(vdc ref), Scope/1, Out Bus Element4/1
  vdc1/1 -> DC voltage controller & current reference/4(vdc)
  vabc (pu)/1 -> PLL & Measurements/1(V)
  PLL & Measurements/4(Vd) -> [Vd], Scope1/1, Out Bus Element5/1
  PLL & Measurements/1(mag) -> Scope4/1, [Vmag]
  PLL & Measurements/3(Vq) -> [Vq], Scope1/2, Out Bus Element6/1
  Product/1 -> DC voltage controller & current reference/3(P pv)
  vdc (V)/1 -> Product/2, Out Bus Element1/1
  Qref (pu)/1 -> DC voltage controller & current reference/1(Q ref)
  DC voltage controller & current reference/2(id ref) -> [id_ref], Out Bus Element3/1
  DC voltage controller & current reference/1(iq ref) -> [iq_ref], Out Bus Element2/1
  [Vd] -> DC voltage controller & current reference/2(Vmag)
  iabc (pu)/1 -> Park Transform1/1
  [ipvd] -> Scope2/2, Current_controller/2(ipvd)
  [theta] -> Inverse Park Transform1/2
  [theta] -> Park Transform1/2
  [ipvq] -> Scope3/2, Current_controller/4(iq)
  [iq_ref] -> Scope3/1, Current_controller/3(iqref)
  [Vd] -> Scope6/1, Current_controller/5(Vd)
  [id_ref] -> Scope2/1, Current_controller/1(id-ref)
  Park Transform1/1 -> Demux1/1
  [vdq0Ref] -> Scope5/1, Inverse Park Transform1/1
  Demux1/3 -> Terminator1/1
  Demux1/1 -> [ipvd], Out Bus Element7/1
  Inverse Park Transform1/1 -> vabcRef (pu)/1
  Demux1/2 -> [ipvq], Out Bus Element8/1
  Current_controller/1(Refrence_mdq0) -> [vdq0Ref]
  [Vq] -> Scope6/2, Current_controller/6(Vq)

== system Nanogrid/Solar Plant Integrated/Detailed/PV Plant & Controller/Controller/Power Reference/Power Reference Controller ==
  Iabc : Inport
  Vabc : Inport  Port=2
  Pref : Inport  Port=3
  Qref : Inport  Port=4
  Constant : Constant  Value=10
  PLL & Measurements : Subsystem
      mask Display: image('$imagefile'); % Use "Edit Image" on toolstrip to change.
  Power Reference Controller : Subsystem  mask{mp=0, mv=0, P=Real power, MVA=MVA, zbase=Vac^2/(MVA), L=L, Imax=Imax, Td=1e-3, Kpic=Kpic, Kiic=Kiic, Kd=0}
      mask prompts: mp "Real power droop cofficient"; mv "Reactive power droop cofficient"; P "Priority mode"; MVA "Base Power (V*A)"; zbase "Base Impedance (Ohm)"; L "Filter Inductance (H)"; Imax "Inverter current limit (pu)"; Td "Sensor time delay (s)"; Kpic "Proportional gain"; Kiic "Integral gain"; Kd "Derevative gain"
      mask TypeOptions P: Real power  | Reactive power
      mask DialogControl Container4 Prompt: General
      mask DialogControl Container5 Prompt: Current Controller
  mabc : Outport
  wires:
  Pref/1 -> Power Reference Controller/3(Pref)
  PLL & Measurements/1(VIbus) -> Power Reference Controller/1(VIbus)
  Power Reference Controller/1(m_abc) -> mabc/1
  Iabc/1 -> PLL & Measurements/2(I)
  Vabc/1 -> PLL & Measurements/1(V)
  Constant/1 -> Power Reference Controller/2(LVRT_iq)
  Qref/1 -> Power Reference Controller/4(Qref)

== system Nanogrid/Solar Plant Integrated/Detailed/PV Plant & Controller/PV Plant/Converter/Average ==
  mabc : Inport
  Converter : ee_lib/Semiconductors & Converters/Converters/Average-Value Voltage Source Converter (Three-Phase)  port_option=ee.enum.threePhasePort.composite  enable_block_pulses_input=false  krec=0.01 Ohm  frequency_option=ee.enum.converters.frequency.variable  input_option=ee.enum.converters.inputOption.ModWave  FRated=60 Hz  losses_parameterization=ee.enum.converters.losses.fixed  Pfixed=0.5 W  ks=0.01  kc1=1.7 V  kc2=0.01 Ohm  Ploss_vect=[100, 800, 1870, 3250, 4900] W  Irms_vect=[10, 100, 200, 300, 400] A  Vdc_nom=300 V  thermal_mass=30000 J/K  temperature_specify=off  temperature_priority=High  temperature=298.15 K  temperature_nominal_specify=off  temperature_nominal_value=1  temperature_nominal_unit=K
  Simulink-PS Converter : nesl_utility/Simulink-PS Converter  PhysicalDomain=network_engine_domain  SubClassName=ps_input  LeftPortType=input  RightPortType=output  PseudoPeriodic=off  Frequencies=[]  NoiseDistribution=none  NoiseParameters=[]  Unit=1  AffineConversion=off  FilteringAndDerivatives=provide  SimscapeFilterOrder=1  InputFilterTimeConstant=0.001  UdotUserProvided=0
  + : PMIOPort  Side=Left
  - : PMIOPort  Port=2  Side=Left
  ~ : PMIOPort  Port=3  Side=Right
  wires:
  mabc/1 -> Simulink-PS Converter/1
  connections:
  Simulink-PS Converter/RConn1 -- Converter/LConn1
  ~/RConn1 -- Converter/LConn2
  -/RConn1 -- Converter/RConn2
  +/RConn1 -- Converter/RConn1

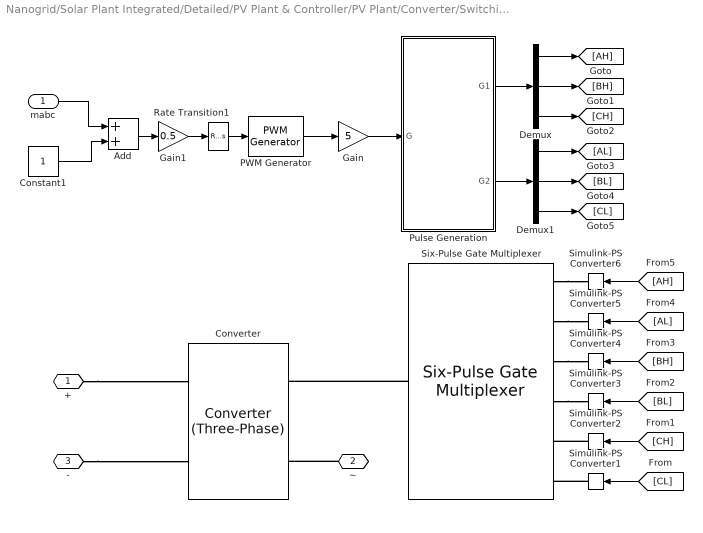
== system Nanogrid/Solar Plant Integrated/Detailed/PV Plant & Controller/PV Plant/Converter/Switching ==
  mabc : Inport
  Add : Sum
  Constant1 : Constant
  Converter : ee_lib/Semiconductors & Converters/Converters/Converter (Three-Phase)  port_option=ee.enum.threePhasePort.composite  fidelity_option=ee.enum.converters.fidelity.detailed  device_type=ee.enum.converters.switchingdevice.ideal  showThermalPort=false  K=0  Vth=1 V  Vgt=1 V  Vgt_off=-1 V  Ih=1 A  Vf=0.8 V  Ron=0.001 Ohm  Rds=0.001 Ohm  Goff=1e-6 1/Ohm  Eon_scalar=22.86e-3 J  Eoff_scalar=17.14e-3 J  Eoff_natural_commutation=10e-3 J  Voff=300 V  Iout_scalar=600 A  onCurrentMeasDelay=0 s  useCurrentFromPreviousCycle=false  useVoltageFromPreviousCycle=false  diode_param=ee.enum.converters.protectiondiode.nodynamics  diode_Vf=0.01 V  diode_Ron=0.0001 Ohm  diode_Goff=1e-5 1/Ohm  diode_C=50 nF  diode_iRM=-235 A  diode_iF=300 A  diode_idot=-50 A/us  diode_trr_param=ee.enum.converters.diodetrr.trr_factor  diode_trr_factor=3  diode_trr=15 us  diode_Qrr=1500 s*uA  diode_rec_loss_model=ee.enum.diode.reverseRecoveryModel.fixed  diode_ErecVal=0 J  diode_scaleWithIandV=false  diode_ErecMat=zeros(2, 3) J  diode_TjrecVec=[298.15, 398.15] K  diode_IfrecVec=[.1, 1, 10] A  diode_IrecVal=10 A  diode_VrecVal=10 V  diode_tFilter=1 / 1000 / 100 s  thermal_network_parameterization=ee.enum.thermalNetworkTopology.external  Rth=[.08, .5] K/W  Rth_Cauer=[.08, .1, .5] K/W  Rth_Foster=[.08, .14, .22, .16] K/W  thermal_mass_parameterization=ee.enum.thermalNetwork.timeconstant  thermal_mass=[.01, .5] J/K  thermal_mass_Cauer=[.01, .1, .5] J/K  thermal_mass_Foster=[.001, .005, .05, .5] J/K  thermal_time_constant=[.001, .2] s  thermal_time_constant_Cauer=[.001, .1, .2] s  thermal_time_constant_Foster=[7e-05, .0007, .01, .08] s  thermal_mass_initial_temperatures=[25, 25] degC  thermal_mass_initial_temperatures_Cauer=[25, 25, 25] degC  junction_thermal_mass=0.01 J/K  Tvec_initial_Foster=[25, 25, 25, 25] degC  snubber_type=ee.enum.converters.snubber.exclude  Cs=1e-7 F  Rs=0.1 Ohm  Vce_loss=[0, 150, 300] V
  Demux : Demux  Outputs=3
  Demux1 : Demux  Outputs=3
  Gain : Gain  Gain=5
  Gain1 : Gain  Gain=0.5
  PWM Generator : eePwmGenerator/PWM Generator  CarrCount=Up  Tper=1/(fSw*1000)  Tdelay=0  Ts=1/(10*fSw*1000)
  Pulse Generation : Subsystem
  Rate Transition1 : RateTransition  OutPortSampleTime=1/(10*fSw*1000)
  Simulink-PS Converter{1..6} (6 alike) : nesl_utility/Simulink-PS Converter  PhysicalDomain=network_engine_domain  SubClassName=ps_input  LeftPortType=input  RightPortType=output  PseudoPeriodic=off  Frequencies=[]  NoiseDistribution=none  NoiseParameters=[]  Unit=1  AffineConversion=off  FilteringAndDerivatives=provide  SimscapeFilterOrder=1  InputFilterTimeConstant=0.001  UdotUserProvided=0
  Six-Pulse Gate Multiplexer : ee_lib/Semiconductors & Converters/Converters/Six-Pulse Gate Multiplexer  port_option=ee.enum.controlport.ps
  + : PMIOPort  Side=Left
  ~ : PMIOPort  Port=2  Side=Right
  - : PMIOPort  Port=3  Side=Left
  wires:
  Demux1/1 -> [AL]
  [BL] -> Simulink-PS Converter3/1
  [AH] -> Simulink-PS Converter6/1
  Demux1/3 -> [CL]
  Gain1/1 -> Rate Transition1/1
  Demux/3 -> [CH]
  Demux/2 -> [BH]
  [CL] -> Simulink-PS Converter1/1
  Constant1/1 -> Add/2
  Add/1 -> Gain1/1
  Gain/1 -> Pulse Generation/1(G)
  PWM Generator/1 -> Gain/1
  mabc/1 -> Add/1
  [CH] -> Simulink-PS Converter2/1
  [AL] -> Simulink-PS Converter5/1
  Demux1/2 -> [BL]
  Demux/1 -> [AH]
  Rate Transition1/1 -> PWM Generator/1
  Pulse Generation/2(G2) -> Demux1/1
  Pulse Generation/1(G1) -> Demux/1
  [BH] -> Simulink-PS Converter4/1
  connections:
  ~/RConn1 -- Converter/LConn2
  Six-Pulse Gate Multiplexer/LConn2 -- Simulink-PS Converter5/RConn1
  Simulink-PS Converter2/RConn1 -- Six-Pulse Gate Multiplexer/LConn5
  Simulink-PS Converter1/RConn1 -- Six-Pulse Gate Multiplexer/LConn6
  Six-Pulse Gate Multiplexer/LConn3 -- Simulink-PS Converter4/RConn1
  Six-Pulse Gate Multiplexer/RConn1 -- Converter/LConn1
  Six-Pulse Gate Multiplexer/LConn1 -- Simulink-PS Converter6/RConn1
  Six-Pulse Gate Multiplexer/LConn4 -- Simulink-PS Converter3/RConn1
  +/RConn1 -- Converter/RConn1
  -/RConn1 -- Converter/RConn2

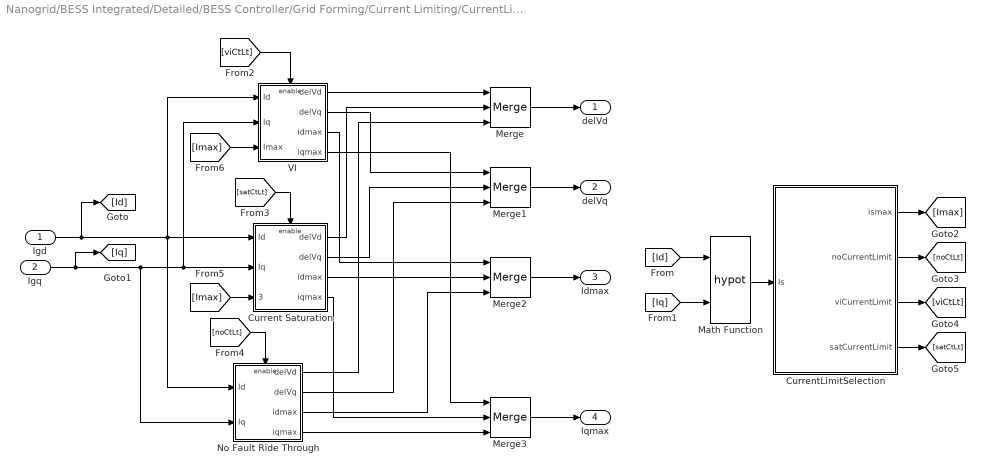
== system Nanogrid/BESS Integrated/Detailed/BESS Controller/Grid Forming/Current Limiting/CurrentLimitingMethod/currentLimitAndVirtual ==
  Igd : Inport
  Igq : Inport  Port=2
  Current Saturation : Subsystem
  CurrentLimitSelection : Stateflow chart  TreatAsAtomicUnit=on
  Math Function : Math  Operator=hypot
  Merge{,1..3} (4 alike) : Merge  Inputs=3
  No Fault Ride Through : Subsystem
  VI : Subsystem
  delVd : Outport
  delVq : Outport  Port=2
  Idmax : Outport  Port=3
  Iqmax : Outport  Port=4
  wires:
  [Imax] -> VI/3(Imax)
  [Imax] -> Current Saturation/3(Imaxsat)
  [noCtLt] -> No Fault Ride Through/Enable
  [satCtLt] -> Current Saturation/Enable
  [viCtLt] -> VI/Enable
  CurrentLimitSelection/4(satCurrentLimit) -> [satCtLt]
  CurrentLimitSelection/3(viCurrentLimit) -> [viCtLt]
  CurrentLimitSelection/2(noCurrentLimit) -> [noCtLt]
  CurrentLimitSelection/1(ismax) -> [Imax]
  Math Function/1 -> CurrentLimitSelection/1(Is)
  No Fault Ride Through/2(delVq) -> Merge1/3
  Merge3/1 -> Iqmax/1
  Current Saturation/2(delVq) -> Merge1/2
  No Fault Ride Through/4(iqmax) -> Merge3/3
  VI/3(idmax) -> Merge2/1
  VI/4(iqmax) -> Merge3/1
  Current Saturation/3(idmax) -> Merge2/2
  VI/2(delVq) -> Merge1/1
  Merge/1 -> delVd/1
  Current Saturation/4(iqmax) -> Merge3/2
  Current Saturation/1(delVd) -> Merge/2
  [Id] -> Math Function/1
  [Iq] -> Math Function/2
  VI/1(delVd) -> Merge/1
  No Fault Ride Through/3(idmax) -> Merge2/3
  No Fault Ride Through/1(delVd) -> Merge/3
  Igd/1 -> [Id], No Fault Ride Through/1(Id), Current Saturation/1(Id), VI/1(Id)
  Merge1/1 -> delVq/1
  Igq/1 -> [Iq], No Fault Ride Through/2(Iq), VI/2(Iq), Current Saturation/2(Iq)
  Merge2/1 -> Idmax/1

== system Nanogrid/BESS Integrated/Detailed/BESS Controller/Grid Forming/Current Limiting/CurrentLimitingMethod/currentSaturation ==
  note: Vs-delV
  Igd : Inport
  Igq : Inport  Port=2
  Compare : Subsystem
  Constant : Constant  Value=maxSatCurrentLimit
  Constant1 : Constant  Value=0
  Constant2 : Constant  Value=0
  If : If
  If Action Subsystem : Subsystem  TreatAsAtomicUnit=on
  If Action Subsystem1 : Subsystem  TreatAsAtomicUnit=on
  Math Function : Math  Operator=hypot
  Merge : Merge
  Merge1 : Merge
  Subtract : Sum  Inputs=+-
  delVd : Outport
  delVq : Outport  Port=2
  Idmax : Outport  Port=3
  Iqmax : Outport  Port=4
  wires:
  Merge1/1 -> Iqmax/1
  Merge/1 -> Idmax/1
  Constant1/1 -> delVd/1
  Constant2/1 -> delVq/1
  If Action Subsystem1/2(Iqmax) -> Merge1/2
  If Action Subsystem/2(Iqmax) -> Merge1/1
  If Action Subsystem1/1(Idmax) -> Merge/2
  If Action Subsystem/1(Idmax) -> Merge/1
  [Is] -> If Action Subsystem/1(Is)
  If/2 -> If Action Subsystem1/Action
  Compare/1(Out1) -> If/1
  Subtract/1 -> Compare/1(u)
  [Isq] -> If Action Subsystem/3(Isq)
  [Isd] -> If Action Subsystem/2(Isd)
  If/1 -> If Action Subsystem/Action
  Math Function/1 -> Subtract/2, [Is]  "Is"
  Constant/1 -> Subtract/1
  Igq/1 -> Math Function/2, [Isq]
  Igd/1 -> Math Function/1, [Isd]

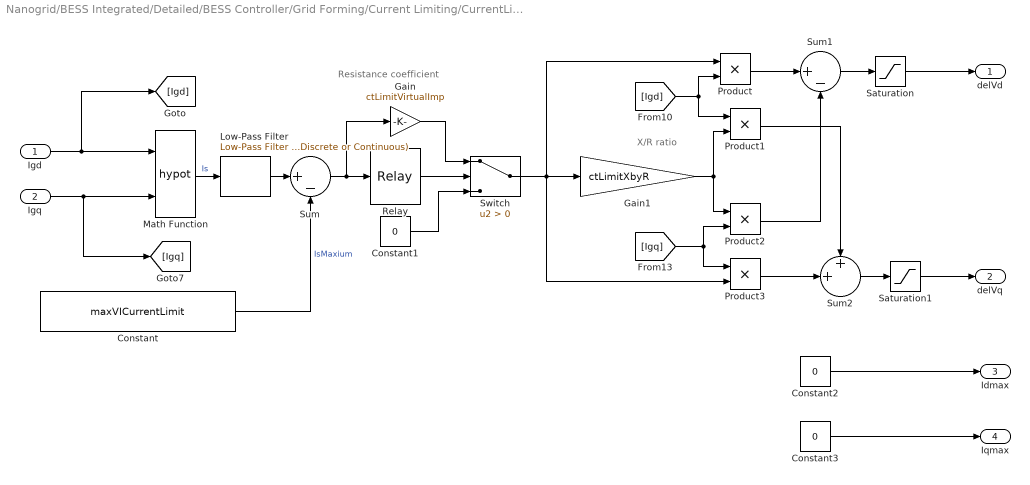
== system Nanogrid/BESS Integrated/Detailed/BESS Controller/Grid Forming/Current Limiting/CurrentLimitingMethod/virtualImpedance ==
  note: Resistance coefficient
  note: X/R ratio
  Igd : Inport
  Igq : Inport  Port=2
  Constant : Constant  Value=maxVICurrentLimit
  Constant1 : Constant  Value=0
  Constant2 : Constant  Value=0
  Constant3 : Constant  Value=0
  Gain : Gain  Gain=ctLimitVirtualImp
  Gain1 : Gain  Gain=ctLimitXbyR
  Low-Pass Filter : eeGeneralControl/Low-Pass Filter (Discrete or Continuous)  K=1  T=currentVITimeConst  B=inf  A=-inf  init_option=Inherited from block input  x0=0  Ts=-1
  Math Function : Math  Operator=hypot
  Product{,1..3} (4 alike) : Product
  Relay : Relay  OnSwitchValue=0.01  OffSwitchValue=-0.05
  Saturation : Saturate  UpperLimit=1  LowerLimit=-1
  Saturation1 : Saturate  UpperLimit=1  LowerLimit=-1
  Sum : Sum  Inputs=|+-
  Sum1 : Sum  Inputs=|+-
  Sum2 : Sum  Inputs=++|
  Switch : Switch  Criteria=u2 > Threshold  SaturateOnIntegerOverflow=off  InputSameDT=off
  delVd : Outport
  delVq : Outport  Port=2
  Idmax : Outport  Port=3
  Iqmax : Outport  Port=4
  wires:
  Sum2/1 -> Saturation1/1
  Product3/1 -> Sum2/2
  Low-Pass Filter/1 -> Sum/1
  Saturation/1 -> delVd/1
  Relay/1 -> Switch/2
  Saturation1/1 -> delVq/1
  Igd/1 -> [Igd], Math Function/1
  Constant1/1 -> Switch/3
  Gain/1 -> Switch/1
  Constant3/1 -> Iqmax/1
  Constant2/1 -> Idmax/1
  [Igd] -> Product/2, Product1/1
  Switch/1 -> Product/1, Product3/2, Gain1/1
  [Igq] -> Product2/2, Product3/1
  Math Function/1 -> Low-Pass Filter/1  "Is"
  Constant/1 -> Sum/2  "IsMaxium"
  Product2/1 -> Sum1/2
  Product/1 -> Sum1/1
  Sum1/1 -> Saturation/1
  Gain1/1 -> Product2/1, Product1/2
  Product1/1 -> Sum2/1
  Igq/1 -> Math Function/2, [Igq]
  Sum/1 -> Relay/1, Gain/1

== system Nanogrid/BESS Integrated/Detailed/BESS Controller/Grid Forming/Grid Voltage Reactive Power Support/Modifying Active Power Reference/Computing New Active Power Ref ==
  Iq : Inport
  Vd : Inport  Port=2
  Abs : Abs  SaturateOnIntegerOverflow=off
  Constant : Constant  Value=maxVICurrentLimit*0.96
  Constant1 : Constant  Value=0
  Product : Product
  Sqrt : Sqrt
  Square : Math  Operator=square
  Square1 : Math  Operator=square
  Subtract : Sum  Inputs=-+
  Switch : Switch  Criteria=u2 > Threshold  Threshold=1.15  SaturateOnIntegerOverflow=off  InputSameDT=off
  Pref : Outport
  wires:
  Product/1 -> Pref/1
  Iq/1 -> Square/1
  Sqrt/1 -> Abs/1
  Vd/1 -> Product/1
  Constant1/1 -> Switch/1
  Square1/1 -> Subtract/2
  Square/1 -> Switch/2, Subtract/1
  Switch/1 -> Product/2
  Subtract/1 -> Sqrt/1
  Constant/1 -> Square1/1
  Abs/1 -> Switch/3

== system Nanogrid/BESS Integrated/Detailed/BESS Controller/Grid Forming/Grid Voltage Reactive Power Support/Modifying Reactive Power Reference/Changing the Power Reference ==
  Vs : Inport
  Vd : Inport  Port=2
  Pref : Inport  Port=3
  Qref : Inport  Port=4
  Enable : EnablePort
  ActivePowerReference : Subsystem
  Constant1 : Constant  Value=voltreference*0.96
  EstimateIdForGivenIq : Subsystem
  EstimateIqForReactivePower : Subsystem
  Max : MinMax  Function=max  Inputs=2
  ReactivePowerReference : Subsystem
  Prefv : Outport
  Qrefv : Outport  Port=2
  wires:
  Vd/1 -> EstimateIqForReactivePower/2(Vd)
  Qref/1 -> Max/2
  ReactivePowerReference/1(QrefNew) -> Max/1
  Pref/1 -> ActivePowerReference/3(Pref)
  EstimateIdForGivenIq/1(Id) -> ActivePowerReference/1(Id)
  Vs/1 -> ReactivePowerReference/1(Vd), EstimateIqForReactivePower/3(Vs), ActivePowerReference/2(Vd)
  Constant1/1 -> EstimateIqForReactivePower/1(Vmin)
  EstimateIqForReactivePower/1(Iq) -> ReactivePowerReference/2(Iq), EstimateIdForGivenIq/1(Iq)
  Max/1 -> Qrefv/1
  ActivePowerReference/1(PrefNew) -> Prefv/1

== system Nanogrid/BESS Integrated/Detailed/BESS Controller/Grid Forming/Grid Voltage Reactive Power Support/Modifying Reactive Power Reference/Hysteresis ==
  Vs : Inport
  AND : Logic  IconShape=distinctive  AllPortsSameDT=off  OutDataTypeStr=boolean
  Compare To Constant : simulink/Logic and Bit Operations/Compare To Constant  relop=<  const=0.9  OutDataTypeStr=boolean
  Compare To Constant1 : simulink/Logic and Bit Operations/Compare To Constant  relop=<  const=0.95  OutDataTypeStr=boolean
  D Latch : simulink_extras/Flip Flops/D Latch
  OR : Logic  Operator=OR  IconShape=distinctive  AllPortsSameDT=off  OutDataTypeStr=boolean
  Scope : Scope
      settings: ActiveDisplayYMinimum=0.96929  ActiveDisplayYMaximum=1.01111
  Terminator : Terminator
  LVFlag : Outport
  wires:
  Vs/1 -> Compare To Constant/1, Compare To Constant1/1, Scope/1
  Compare To Constant/1 -> OR/2, D Latch/2, D Latch/1
  D Latch/2 -> Terminator/1
  OR/1 -> LVFlag/1
  AND/1 -> OR/1
  D Latch/1 -> AND/2
  Compare To Constant1/1 -> AND/1

== system Nanogrid/BESS Integrated/Detailed/BESS Controller/Grid Forming/Grid Voltage Reactive Power Support/Modifying Reactive Power Reference/Not Altering the Power Reference ==
  Pref : Inport
  Qref : Inport  Port=2
  Enable : EnablePort
  Prefv : Outport
  Qrefv : Outport  Port=2
  wires:
  Qref/1 -> Qrefv/1
  Pref/1 -> Prefv/1
